simulink subsystem "CircuitBreaker"  (R2023b)
settings: Solver=VariableStepAuto  StartTime=0.0  StopTime=10.0  RelTol=1e-3
undefined symbols (not defined in the file): f
libraries: spsThreePhaseBreakerLib x1, instrumentlib x1
settings Model: Creator=javiersanderios  LastModifiedBy=javiersanderios

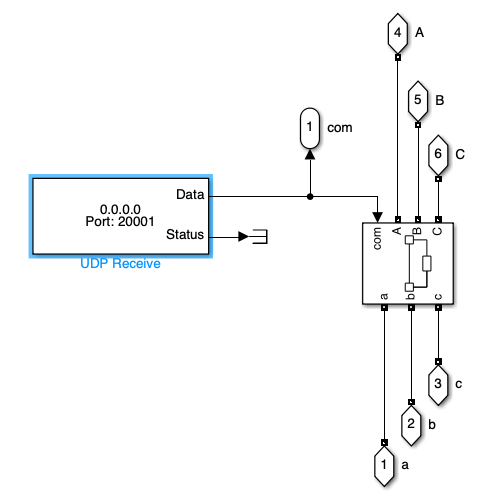
[thumbnail: Simulink's stored preview of the top-level diagram]
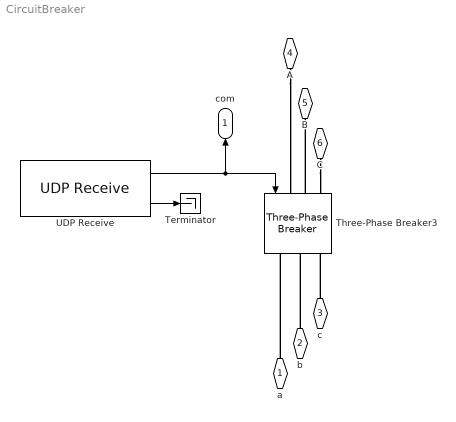
== system CircuitBreaker ==
  Terminator : Terminator
  Three-Phase Breaker3 : spsThreePhaseBreakerLib/Three-Phase Breaker  InitialState=closed  SwitchA=on  SwitchB=on  SwitchC=on  SwitchTimes=[0.2]  External=on  BreakerResistance=0.01  SnubberResistance=1e6  SnubberCapacitance=inf  Measurements=Breaker voltages and currents
  UDP Receive : instrumentlib/UDP Receive  LocalAddress=0.0.0.0  LocalPort=20001  EnablePortSharing=off  Host=10.0.1.2  Port=20001  GetLatestData=off  DataSize=[ 1, 1 ]  DataType=uint16  ASCIIFormatting=%f,  Terminator=LF  CustomTerminator=10  ByteOrder=big-endian  EnableBlockingMode=off  Timeout=10  SampleTime=0.01  SimulateUsing=Interpreted execution
  a : PMIOPort  Side=Left
  b : PMIOPort  Port=2  Side=Left
  c : PMIOPort  Port=3  Side=Left
  A : PMIOPort  Port=4  Side=Right
  B : PMIOPort  Port=5  Side=Right
  C : PMIOPort  Port=6  Side=Right
  com : Outport
  wires:
  UDP Receive/1 -> Three-Phase Breaker3/1, com/1
  UDP Receive/2 -> Terminator/1
  connections:
  b/RConn1 -- Three-Phase Breaker3/RConn2
  c/RConn1 -- Three-Phase Breaker3/RConn3
  A/RConn1 -- Three-Phase Breaker3/LConn1
  Three-Phase Breaker3/LConn2 -- B/RConn1
  C/RConn1 -- Three-Phase Breaker3/LConn3
  a/RConn1 -- Three-Phase Breaker3/RConn1
